simulink model "model8_streaming_qpsk_ofdm_no_pluto"  (R2025b)
settings: Solver=VariableStepAuto  StartTime=0.0  StopTime=10.0  RelTol=1e-3
values from neighbouring files (symbols this model uses):
  preambleBits = repmat(basePattern, 12, 1)    [setup_simulink_streaming.m]    (also in setup_simulink_streaming_3sym_uncoded.m; setup_simulink_streaming_coded_const.m)
  txPayloadBits = randi([0 1], payloadBitsPerFrame, 1)    [setup_simulink_streaming.m]    (also in setup_simulink_streaming_3sym_uncoded.m; setup_simulink_streaming_coded_const.m)
libraries: commofdm x2, commdigbbndpm3 x2, commchan3 x1
settings Model: Creator=Naren  LastModifiedBy=Naren

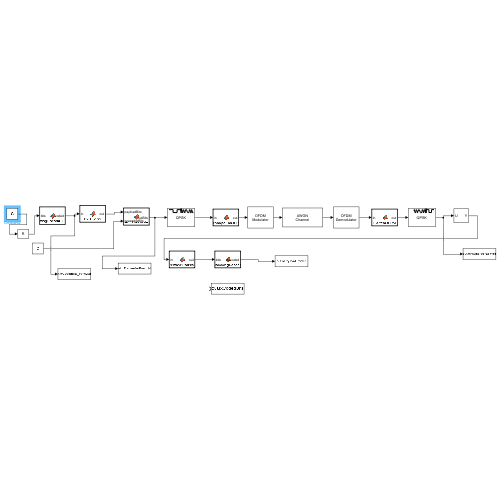
[thumbnail: Simulink's stored preview of the top-level diagram]
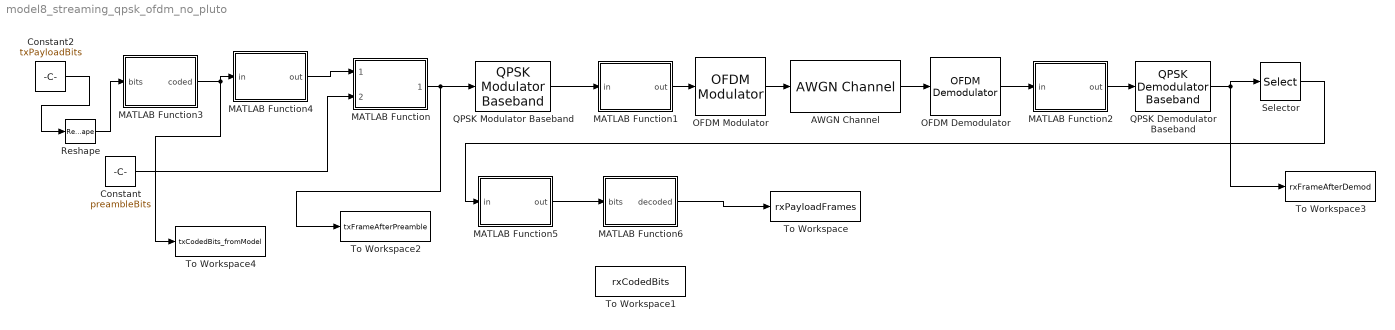
== system model8_streaming_qpsk_ofdm_no_pluto ==
  AWGN Channel : commchan3/AWGN Channel  LegacyMode=off  NoiseMethod="Signal to noise ratio  (SNR)"  noiseMode="Signal to noise ratio  (SNR)"  EbNo=10  EsNo=10  SNR=10  BitsPerSymbol=1  SignalPower=1  SpecifySymbolPeriod=off  SamplesPerSymbol=1  SymbolPeriod=1  VarianceSource=Parameter  Variance=1  RandomStream=Global stream  Seed=67  SimulateUsing=Code generation
  Constant : Constant  Value=preambleBits  SampleTime=1
  Constant2 : Constant  Value=txPayloadBits  VectorParams1D=off  SampleTime=1
  MATLAB Function : MATLAB Function  TreatAsAtomicUnit=on
  MATLAB Function1 : MATLAB Function  TreatAsAtomicUnit=on
  MATLAB Function2 : MATLAB Function  TreatAsAtomicUnit=on
  MATLAB Function3 : MATLAB Function  TreatAsAtomicUnit=on
  MATLAB Function4 : MATLAB Function  TreatAsAtomicUnit=on
  MATLAB Function5 : MATLAB Function  TreatAsAtomicUnit=on
  MATLAB Function6 : MATLAB Function  TreatAsAtomicUnit=on
  OFDM Demodulator : commofdm/OFDM Demodulator  StatePerturbationForJacobian=1.0e-05  FFTLength=64  NumGuardBandCarriers=[8; 7]  RemoveDCCarrier=on  PilotOutputPort=off  PilotCarrierIndices=[12; 26; 40; 54]  CyclicPrefixLength=16  OversamplingFactor=1  NumSymbols=3  NumReceiveAntennas=1  SimulateUsing=Interpreted execution
  OFDM Modulator : commofdm/OFDM Modulator  StatePerturbationForJacobian=1.0e-05  FFTLength=64  NumGuardBandCarriers=[8; 7]  InsertDCNull=on  PilotInputPort=off  PilotCarrierIndices=[12; 26; 40; 54]  CyclicPrefixLength=16  Windowing=off  WindowLength=1  OversamplingFactor=1  NumSymbols=3  NumTransmitAntennas=1  SimulateUsing=Interpreted execution
  QPSK Demodulator Baseband : commdigbbndpm3/QPSK Demodulator Baseband  OutType=Bit  DecType=Hard decision  VarSource=Dialog  Variance=1  Dec=Gray  Ph=pi/4  outDtype1=Inherit via internal rule  outDtype2=Inherit via internal rule  derotateFactorWordLen=16  derotateFactorDataTypeStr=Inherit: Same word length as input  derotateFactorLastDataTypeStr=Inherit: Same word length as input
  QPSK Modulator Baseband : commdigbbndpm3/QPSK Modulator Baseband  InType=Bit  Enc=Gray  Ph=pi/4  outDtype=double  outWordLen=16  outUDDataType=sfix(16)  outFracLenMode=Best precision  outFracLen=15  outDataTypeStr=double  outLastDataTypeStr=double
  Reshape : Reshape  OutputDimensionality=Customize  OutputDimensions=[96 1]
  Selector : Selector  InputPortWidth=288  IndexOptions=Index vector (dialog)  Indices=97:288  OutputSizes=1
  To Workspace : ToWorkspace  VariableName=rxPayloadFrames  SampleTime=-1
  To Workspace1 : ToWorkspace  VariableName=rxCodedBits  SampleTime=-1
  To Workspace2 : ToWorkspace  VariableName=txFrameAfterPreamble  SampleTime=-1
  To Workspace3 : ToWorkspace  VariableName=rxFrameAfterDemod  SampleTime=-1
  To Workspace4 : ToWorkspace  VariableName=txCodedBits_fromModel  SampleTime=-1
  wires:
  Constant/1 -> MATLAB Function/2(preambleBits)
  MATLAB Function/1(outBits) -> QPSK Modulator Baseband/1, To Workspace2/1
  QPSK Modulator Baseband/1 -> MATLAB Function1/1(in)
  MATLAB Function1/1(out) -> OFDM Modulator/1
  OFDM Demodulator/1 -> MATLAB Function2/1(in)
  MATLAB Function2/1(out) -> QPSK Demodulator Baseband/1
  QPSK Demodulator Baseband/1 -> Selector/1, To Workspace3/1
  Selector/1 -> MATLAB Function5/1(in)
  MATLAB Function3/1(coded) -> MATLAB Function4/1(in), To Workspace4/1
  MATLAB Function4/1(out) -> MATLAB Function/1(payloadBits)
  OFDM Modulator/1 -> AWGN Channel/1
  AWGN Channel/1 -> OFDM Demodulator/1
  MATLAB Function5/1(out) -> MATLAB Function6/1(bits)
  MATLAB Function6/1(decoded) -> To Workspace/1
  Constant2/1 -> Reshape/1
  Reshape/1 -> MATLAB Function3/1(bits)

== matlab function model8_streaming_qpsk_ofdm_no_pluto/MATLAB Function ==
  data: payloadBits input; outBits output; preambleBits input
function outBits = AddPreamble(payloadBits, preambleBits)
%#codegen

outBits = zeros(288,1);
outBits(1:96) = preambleBits;
outBits(97:288) = payloadBits;

== matlab function model8_streaming_qpsk_ofdm_no_pluto/MATLAB Function2 ==
  data: in input; out output
function out = FlattenOFDM(in)
%#codegen

out = complex(zeros(144,1));
out(:) = in(:);

== matlab function model8_streaming_qpsk_ofdm_no_pluto/MATLAB Function3 ==
  data: bits input; coded output
function coded = HammingEncode_FIXED(bits)
%#codegen

% Force correct shape
bits = reshape(bits, 96, 1);

coded = zeros(168,1);

for k = 1:24
    idxIn = 4*(k-1) + 1;

    d1 = bits(idxIn);
    d2 = bits(idxIn+1);
    d3 = bits(idxIn+2);
    d4 = bits(idxIn+3);

    p1 = mod(d1 + d2 + d4, 2);
    p2 = mod(d1 + d3 + d4, 2);
    p3 = mod(d2 + d3 + d4, 2);

    idxOut = 7*(k-1) + 1;
    coded(idxOut)   = p1;
    coded(idxOut+1) = p2;
    coded(idxOut+2) = d1;
    coded(idxOut+3) = p3;
    coded(idxOut+4) = d2;
    coded(idxOut+5) = d3;
    coded(idxOut+6) = d4;
end

== matlab function model8_streaming_qpsk_ofdm_no_pluto/MATLAB Function4 ==
  data: in input; out output
function out = PadTo192(in)
%#codegen

out = zeros(192,1);
out(1:168) = in;

== matlab function model8_streaming_qpsk_ofdm_no_pluto/MATLAB Function5 ==
  data: in input; out output
function out = RemovePad168(in)
%#codegen

out = zeros(168,1);
out(:) = in(1:168);

== matlab function model8_streaming_qpsk_ofdm_no_pluto/MATLAB Function6 ==
  data: bits input; decoded output
function decoded = HammingDecode(bits)
%#codegen

decoded = zeros(96,1);

for k = 1:24
    idxIn = 7*(k-1) + 1;

    cw1 = bits(idxIn);
    cw2 = bits(idxIn+1);
    cw3 = bits(idxIn+2);
    cw4 = bits(idxIn+3);
    cw5 = bits(idxIn+4);
    cw6 = bits(idxIn+5);
    cw7 = bits(idxIn+6);

    s1 = mod(cw1 + cw3 + cw5 + cw7, 2);
    s2 = mod(cw2 + cw3 + cw6 + cw7, 2);
    s3 = mod(cw4 + cw5 + cw6 + cw7, 2);

    syndrome = s1 + 2*s2 + 4*s3;

    if syndrome == 1
        cw1 = mod(cw1 + 1, 2);
    elseif syndrome == 2
        cw2 = mod(cw2 + 1, 2);
    elseif syndrome == 3
        cw3 = mod(cw3 + 1, 2);
    elseif syndrome == 4
        cw4 = mod(cw4 + 1, 2);
    elseif syndrome == 5
        cw5 = mod(cw5 + 1, 2);
    elseif syndrome == 6
        cw6 = mod(cw6 + 1, 2);
    elseif syndrome == 7
        cw7 = mod(cw7 + 1, 2);
    end

    idxOut = 4*(k-1) + 1;
    decoded(idxOut)   = cw3;
    decoded(idxOut+1) = cw5;
    decoded(idxOut+2) = cw6;
    decoded(idxOut+3) = cw7;
end

== matlab function model8_streaming_qpsk_ofdm_no_pluto/MATLAB Function1 ==
  data: in input; out output
function out = ReshapeForOFDM(in)
%#codegen

out = complex(zeros(48,3));
out(:) = in(:);

end
